simulink model "Simulador_PID_Velocidad_Motor"  (R2020b)
settings: Solver=FixedStepAuto  StartTime=0.0  StopTime=4  FixedStep=0.02  RelTol=1e-3
libraries: simulink x1
settings Model: Creator=DellXPS13  LastModifiedBy=zunt7
settings DataIOCC: ReturnWorkspaceOutputs=off
settings DebuggingCC: ArithmeticOperatorsInVariantConditions=warning
settings SFSimCC: CustomCodeUndefinedFunction=UseInterfaceOnly

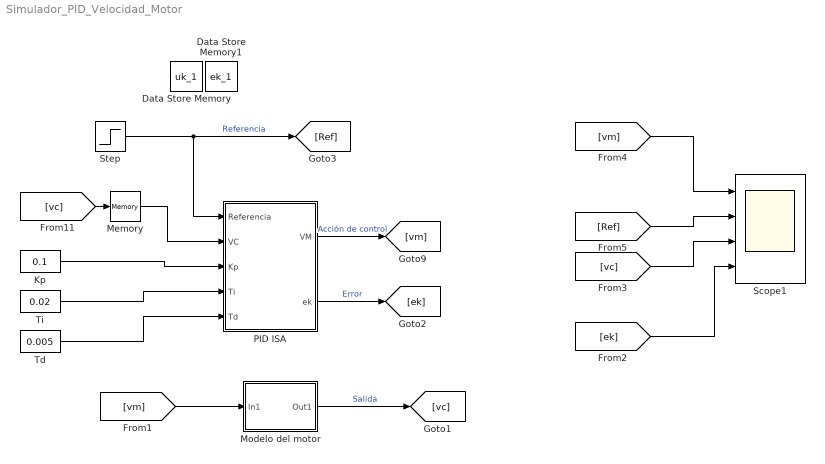
== system Simulador_PID_Velocidad_Motor ==
  Data Store Memory : DataStoreMemory  DataStoreName=uk_1  ReadBeforeWriteMsg=warning  WriteAfterWriteMsg=warning  WriteAfterReadMsg=warning  ShowAdditionalParam=off  OutDataTypeStr=double
  Data Store Memory1 : DataStoreMemory  DataStoreName=ek_1  ReadBeforeWriteMsg=warning  WriteAfterWriteMsg=warning  WriteAfterReadMsg=warning  ShowAdditionalParam=off  OutDataTypeStr=double
  Kp : Constant  Value=0.1
  Memory : Memory  InheritSampleTime=on
  Modelo del motor : Subsystem  mask{k=0.146, tau=0.104, ruido=on}
      mask prompts: k "K (Voltaje medio x k ajuste curva)"; tau "Constante de tiempo (tau)"; ruido "Noise"
  PID ISA : MATLAB Function  TreatAsAtomicUnit=on  SystemSampleTime=0.02
      settings: MinAlgLoopOccurrences=on
  Scope1 : Scope  NumInputPorts=4
  Step : Step  After=10  SampleTime=0
  Td : Constant  Value=0.005
  Ti : Constant  Value=0.02
  wires:
  Kp/1 -> PID ISA/3(Kp)
  Ti/1 -> PID ISA/4(Ti)
  Td/1 -> PID ISA/5(Td)
  PID ISA/1(VM) -> [vm]  "Acción de control"
  [vc] -> Memory/1
  Step/1 -> [Ref], PID ISA/1(Referencia)  "Referencia"
  Memory/1 -> PID ISA/2(VC)
  PID ISA/2(ek) -> [ek]  "Error"
  [vc] -> Scope1/3
  [Ref] -> Scope1/2
  [ek] -> Scope1/4
  [vm] -> Scope1/1
  Modelo del motor/1(Out1) -> [vc]  "Salida"
  [vm] -> Modelo del motor/1(In1)

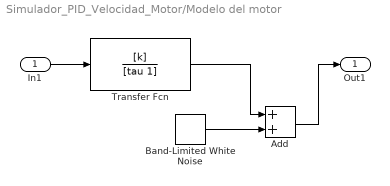
== system Simulador_PID_Velocidad_Motor/Modelo del motor ==
  In1 : Inport
  Add : Sum
  Band-Limited White Noise : simulink/Sources/Band-Limited White Noise  Cov=[0.002]*ruido  Ts=0.02  seed=[23341]
  Transfer Fcn : TransferFcn  Numerator=[k]  Denominator=[tau 1]
  Out1 : Outport  VectorParamsAs1DForOutWhenUnconnected=off
  wires:
  In1/1 -> Transfer Fcn/1
  Transfer Fcn/1 -> Add/1
  Band-Limited White Noise/1 -> Add/2
  Add/1 -> Out1/1

== matlab function Simulador_PID_Velocidad_Motor/PID ISA ==
  data: Referencia input; VM output; VC input; Kp input; Ti input; Td input; uk_1 data_store_memory; ek_1 data_store_memory; ek output
function [VM,ek] = PID(Referencia,VC,Kp,Ti,Td)
Ts = 0.02;
global uk_1 ek_1;

% Calcular el Error COMPLETAR
ek = Referencia - VC ;
% Calcular la Acción de control COMPLETAR
up = Kp * ek;
ui = uk_1 + (Kp/Ti) * ek * Ts;
ud = Kp * Td * ((ek - ek_1) / Ts);

uk =  up + ui + ud;

%Saturar la Acción de Control (-100,+100) COMPLETAR
if (uk >= (100))
    uk = 100;
    ui = uk_1;
end     
if (uk <= (-100))
    uk = -100;
    ui = uk_1;
end

% Sumamos Punto Funcionamiento a la Accion de Control
VM = uk;

% Actualizar variables
uk_1 = ui;
ek_1 = ek;
